simulink model "dtmf"  (R2018b)
settings: Solver=VariableStepAuto  StartTime=0.0  StopTime=105  RelTol=1e-3
libraries: dspsrcs4 x35, simulink x24, dspbuff3 x14, dspsigops x3, dspswit3 x1
settings Model: Creator=sajan.gict16  LastModifiedBy=srg
settings DebuggingCC: LibraryContextMissingDiagnostic=none
settings SFSimCC: SimUseLocalCustomCode=off
settings RTWCC: RTWUseLocalCustomCode=off

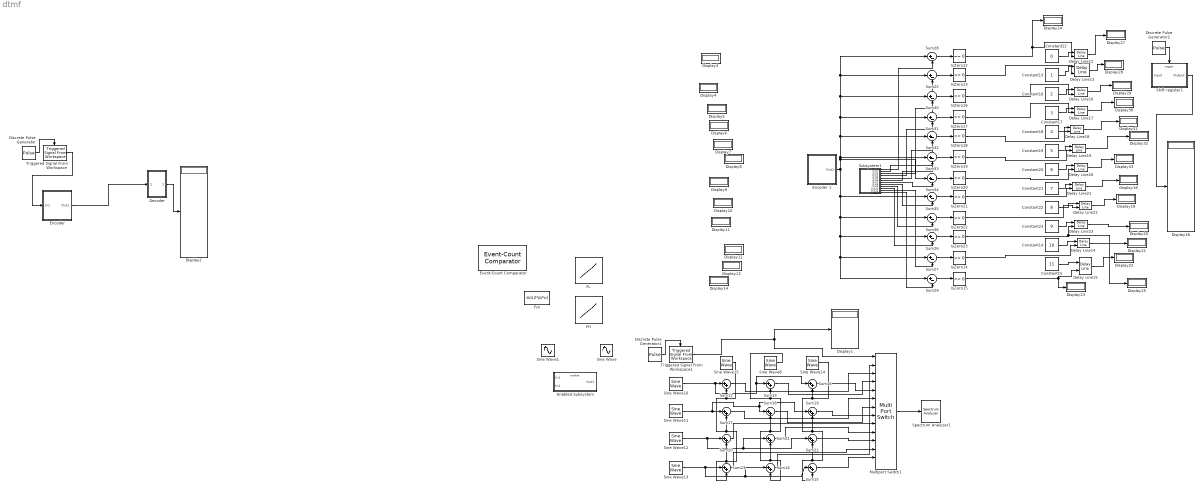
== system dtmf ==
  Constant12 : Constant  Value=0  SampleTime=1/12000
  Constant13 : Constant  SampleTime=1/12000
  Constant14 : Constant  Value=10  SampleTime=1/12000
  Constant15 : Constant  Value=11  SampleTime=1/12000
  Constant16 : Constant  Value=2  SampleTime=1/12000
  Constant17 : Constant  Value=3  SampleTime=1/12000
  Constant18 : Constant  Value=4  SampleTime=1/12000
  Constant19 : Constant  Value=5  SampleTime=1/12000
  Constant20 : Constant  Value=6  SampleTime=1/12000
  Constant21 : Constant  Value=7  SampleTime=1/12000
  Constant22 : Constant  Value=8  SampleTime=1/12000
  Constant23 : Constant  Value=9  SampleTime=1/12000
  "Decoder " : Subsystem
  Delay Line12 : dspbuff3/Delay Line  siz=3  ic=0  directfeed=off  enable_output=on  hold_output=on  OutputFrames=off
      settings: SourceProductName=DSP System Toolbox  SourceProductBaseCode=DS
  Delay Line13 : dspbuff3/Delay Line  siz=2  ic=0  directfeed=off  enable_output=on  hold_output=on  OutputFrames=off
      settings: SourceProductName=DSP System Toolbox  SourceProductBaseCode=DS
  Delay Line14 : dspbuff3/Delay Line  siz=2  ic=0  directfeed=on  enable_output=on  hold_output=on  OutputFrames=off
      settings: SourceProductName=DSP System Toolbox  SourceProductBaseCode=DS
  Delay Line15 : dspbuff3/Delay Line  siz=2  ic=0  directfeed=on  enable_output=on  hold_output=on  OutputFrames=off
      settings: SourceProductName=DSP System Toolbox  SourceProductBaseCode=DS
  Delay Line16 : dspbuff3/Delay Line  siz=3  ic=0  directfeed=off  enable_output=on  hold_output=on  OutputFrames=off
      settings: SourceProductName=DSP System Toolbox  SourceProductBaseCode=DS
  Delay Line17 : dspbuff3/Delay Line  siz=3  ic=0  directfeed=off  enable_output=on  hold_output=off  OutputFrames=off
      settings: SourceProductName=DSP System Toolbox  SourceProductBaseCode=DS
  Delay Line{18..22} (5 alike) : dspbuff3/Delay Line  siz=2  ic=0  directfeed=on  enable_output=on  hold_output=off  OutputFrames=off
      settings: SourceProductName=DSP System Toolbox  SourceProductBaseCode=DS
  Delay Line23 : dspbuff3/Delay Line  siz=2  ic=0  directfeed=off  enable_output=on  hold_output=off  OutputFrames=off
      settings: SourceProductName=DSP System Toolbox  SourceProductBaseCode=DS
  Discrete Pulse Generator : DiscretePulseGenerator  SampleTime=5
  Discrete Pulse Generator1 : DiscretePulseGenerator  SampleTime=5
  Discrete Pulse Generator2 : DiscretePulseGenerator  SampleTime=5
  Display{1..14,18..33} (30 alike) : Display
  Enabled Subsystem : Subsystem  TreatAsAtomicUnit=on
  "Encoder " : Subsystem
  Encoder 1 : Subsystem
  Event-Count Comparator : dspswit3/Event-Count Comparator  Threshold=10
      settings: SourceProductName=DSP System Toolbox  SourceProductBaseCode=DS
  FH : Lookup_n-D  NumberOfTableDimensions=1  BreakpointsForDimension1=[0,1,2,3,4,5,6,7,8,9,10,11]  Table=[1336,1209,1336,1477,1209,1336,1477,1209,1336,1477,1209,1477]  InternalRulePriority=Speed  RndMeth=Simplest  InputSameDT=on
  "FL " : Lookup_n-D  NumberOfTableDimensions=1  BreakpointsForDimension1=[0,1,2,3,4,5,6,7,8,9,10,11]  Table=[941,697,697,697,770,770,770,852,852,852,941,941]  InternalRulePriority=Speed  RndMeth=Simplest  InputSameDT=on
  Fcn : Fcn  Expr=sin(2*pi*u)
  IsZero{12..23} (12 alike) : simulink/Logic and Bit Operations/Compare To Zero  relop===  OutDataTypeStr=boolean
  Multiport Switch1 : MultiPortSwitch  DataPortOrder=Zero-based contiguous  Inputs=12  DataPortIndices={1,2,3,4,5,6,7,8,9,10,0,11}  DataPortForDefault=Additional data port  DiagnosticForDefault=Warning  zeroidx=on
  Shift register1 : Subsystem  TreatAsAtomicUnit=on
  Sine Wave : Sin  SampleTime=0
  Sine Wave1 : Sin  SampleTime=0
  Sine Wave10 : dspsrcs4/Sine Wave  Amplitude=1  Frequency=697  Phase=0  SampleMode=Discrete  OutComplex=Real  CompMethod=Trigonometric fcn  TableSize=Speed  SampleTime=1/12000  SamplesPerFrame=1  ResetState=Restart at time zero  OutputFrames=off  dataType=double  wordLen=16  udDataType=sfix(16)  fracBitsMode=Best precision  numFracBits=15  OutDataTypeStr=double  LastOutDataTypeStr=double
  Sine Wave11 : dspsrcs4/Sine Wave  Amplitude=1  Frequency=770  Phase=0  SampleMode=Discrete  OutComplex=Real  CompMethod=Trigonometric fcn  TableSize=Speed  SampleTime=1/12000  SamplesPerFrame=1  ResetState=Restart at time zero  OutputFrames=off  dataType=double  wordLen=16  udDataType=sfix(16)  fracBitsMode=Best precision  numFracBits=15  OutDataTypeStr=double  LastOutDataTypeStr=double
  Sine Wave12 : dspsrcs4/Sine Wave  Amplitude=1  Frequency=852  Phase=0  SampleMode=Discrete  OutComplex=Real  CompMethod=Trigonometric fcn  TableSize=Speed  SampleTime=1/12000  SamplesPerFrame=1  ResetState=Restart at time zero  OutputFrames=off  dataType=double  wordLen=16  udDataType=sfix(16)  fracBitsMode=Best precision  numFracBits=15  OutDataTypeStr=double  LastOutDataTypeStr=double
  Sine Wave13 : dspsrcs4/Sine Wave  Amplitude=1  Frequency=941  Phase=0  SampleMode=Discrete  OutComplex=Real  CompMethod=Trigonometric fcn  TableSize=Speed  SampleTime=1/12000  SamplesPerFrame=1  ResetState=Restart at time zero  OutputFrames=off  dataType=double  wordLen=16  udDataType=sfix(16)  fracBitsMode=Best precision  numFracBits=15  OutDataTypeStr=double  LastOutDataTypeStr=double
  Sine Wave14 : dspsrcs4/Sine Wave  Amplitude=1  Frequency=1477  Phase=0  SampleMode=Discrete  OutComplex=Real  CompMethod=Trigonometric fcn  TableSize=Speed  SampleTime=1/12000  SamplesPerFrame=1  ResetState=Restart at time zero  OutputFrames=off  dataType=double  wordLen=16  udDataType=sfix(16)  fracBitsMode=Best precision  numFracBits=15  OutDataTypeStr=double  LastOutDataTypeStr=double
  Sine Wave15 : dspsrcs4/Sine Wave  Amplitude=1  Frequency=1209  Phase=0  SampleMode=Discrete  OutComplex=Real  CompMethod=Trigonometric fcn  TableSize=Speed  SampleTime=1/12000  SamplesPerFrame=1  ResetState=Restart at time zero  OutputFrames=off  dataType=double  wordLen=16  udDataType=sfix(16)  fracBitsMode=Best precision  numFracBits=15  OutDataTypeStr=double  LastOutDataTypeStr=double
  Sine Wave8 : dspsrcs4/Sine Wave  Amplitude=1  Frequency=1336  Phase=0  SampleMode=Discrete  OutComplex=Real  CompMethod=Trigonometric fcn  TableSize=Speed  SampleTime=1/12000  SamplesPerFrame=1  ResetState=Restart at time zero  OutputFrames=off  dataType=double  wordLen=16  udDataType=sfix(16)  fracBitsMode=Best precision  numFracBits=15  OutDataTypeStr=double  LastOutDataTypeStr=double
  Spectrum Analyzer1 : SpectrumAnalyzer
  Subsystem1 : Subsystem
  Sum{12..23} (12 alike) : Sum  Inputs=|++
  Sum{25..36} (12 alike) : Sum  Inputs=|+-
  Triggered Signal From Workspace : dspsigops/Triggered Signal From Workspace  Signal=[0 2 0 8 7 6 5 4 9 10]  TriggerType=Rising edge  ic=0  SamplesPerFrame=1  OutputAfterFinalValue=Setting to zero  OutputFrames=off
      settings: SourceProductName=DSP System Toolbox  SourceProductBaseCode=DS
  Triggered Signal From Workspace1 : dspsigops/Triggered Signal From Workspace  Signal=[1 2 3 8 7 6 5 4 9 10]  TriggerType=Rising edge  ic=0  SamplesPerFrame=1  OutputAfterFinalValue=Setting to zero  OutputFrames=off
      settings: SourceProductName=DSP System Toolbox  SourceProductBaseCode=DS
  wires:
  Sum16/1 -> Multiport Switch1/5
  Sum19/1 -> Multiport Switch1/8
  Sum18/1 -> Multiport Switch1/7
  Sum23/1 -> Multiport Switch1/12
  Sine Wave14/1 -> Sum15/2, Sum22/2, Sum19/2, Sum16/2
  Sum15/1 -> Multiport Switch1/13
  Sum21/1 -> Multiport Switch1/10
  Sum12/1 -> Multiport Switch1/3
  Sum17/1 -> Multiport Switch1/6
  Triggered Signal From Workspace1/1 -> Multiport Switch1/1, Display1/1
  Multiport Switch1/1 -> Spectrum Analyzer1/1
  Sum13/1 -> Multiport Switch1/4
  Sine Wave15/1 -> Sum23/2, Sum20/2, Sum17/2, Sum12/2
  Sum20/1 -> Multiport Switch1/9
  Sum14/1 -> Multiport Switch1/2
  Sine Wave8/1 -> Sum14/2, Sum21/2, Sum18/2, Sum13/2
  Sine Wave13/1 -> Sum14/1, Sum15/1, Sum23/1
  Sine Wave11/1 -> Sum18/1, Sum19/1, Sum17/1
  Sine Wave12/1 -> Sum22/1, Sum21/1, Sum20/1
  Sine Wave10/1 -> Sum16/1, Sum13/1, Sum12/1
  Discrete Pulse Generator1/1 -> Triggered Signal From Workspace1/Trigger
  Sum22/1 -> Multiport Switch1/11
  Subsystem1/12(Out12) -> Sum29/2
  Subsystem1/10(Out10) -> Sum26/2
  Subsystem1/9(Out9) -> Sum36/2
  Subsystem1/8(Out8) -> Sum35/2
  Sum28/1 -> IsZero12/1
  IsZero19/1 -> Delay Line19/2
  Constant14/1 -> Delay Line14/1
  IsZero21/1 -> Delay Line21/2
  Subsystem1/4(Out4) -> Sum31/2
  Subsystem1/3(Out3) -> Sum30/2
  Subsystem1/2(Out2) -> Sum25/2
  Subsystem1/7(Out7) -> Sum34/2
  Subsystem1/6(Out6) -> Sum33/2
  Subsystem1/5(Out5) -> Sum32/2
  Sum26/1 -> IsZero23/1
  Sum35/1 -> IsZero21/1
  Sum29/1 -> IsZero15/1
  Sum36/1 -> IsZero22/1
  Sum27/1 -> IsZero14/1
  Subsystem1/1(Out1) -> Sum28/2
  IsZero14/1 -> Delay Line14/2
  Delay Line15/1 -> Display22/1
  Delay Line20/1 -> Display33/1
  Sum31/1 -> IsZero17/1
  Constant18/1 -> Delay Line18/1
  Discrete Pulse Generator2/1 -> Shift register1/Trigger
  IsZero16/1 -> Delay Line16/2
  Encoder 1/1(Out1) -> Sum29/1, Sum27/1, Sum26/1, Sum36/1, Sum35/1, Sum34/1, Sum32/1, Sum28/1, Sum25/1, Sum30/1, Sum31/1, Sum33/1
  IsZero18/1 -> Delay Line18/2
  Sum34/1 -> IsZero20/1
  Delay Line18/1 -> Display31/1
  IsZero20/1 -> Delay Line20/2
  Constant23/1 -> Delay Line23/1
  Constant21/1 -> Delay Line21/1
  IsZero12/1 -> Display24/1, Delay Line12/2
  Delay Line13/1 -> Display28/1
  Constant19/1 -> Delay Line19/1
  IsZero23/1 -> Display25/1, Delay Line23/2
  IsZero13/1 -> Delay Line13/2
  Delay Line14/1 -> Display21/1
  IsZero22/1 -> Delay Line22/2
  IsZero17/1 -> Delay Line17/2
  IsZero15/1 -> Delay Line15/2, Display23/1
  Delay Line21/1 -> Display18/1
  Delay Line22/1 -> Display19/1
  Constant22/1 -> Delay Line22/1
  Delay Line16/1 -> Display29/1
  Constant20/1 -> Delay Line20/1
  Constant17/1 -> Delay Line17/1
  Constant15/1 -> Delay Line15/1
  Constant12/1 -> Delay Line12/1
  Constant16/1 -> Delay Line16/1
  Delay Line17/1 -> Display30/1
  Subsystem1/11(Out11) -> Sum27/2
  Sum32/1 -> IsZero18/1
  Delay Line19/1 -> Display32/1
  Sum30/1 -> IsZero16/1
  Sum25/1 -> IsZero13/1
  Delay Line23/1 -> Display20/1
  Constant13/1 -> Delay Line13/1
  Shift register1/1(Output) -> Display26/1
  Sum33/1 -> IsZero19/1
  Delay Line12/1 -> Display27/1
  ? -> Display6/1
  ? -> Display9/1
  ? -> Display8/1
  ? -> Display10/1
  ? -> Display11/1
  ? -> Display5/1
  ? -> Display12/1
  ? -> Display7/1
  ? -> Display3/1
  ? -> Display14/1
  ? -> Display13/1
  "Encoder "/1(Out1) -> "Decoder "/1(In1)
  "Decoder "/1(Out1) -> Display2/1
  Discrete Pulse Generator/1 -> Triggered Signal From Workspace/Trigger
  Triggered Signal From Workspace/1 -> "Encoder "/1(In1)

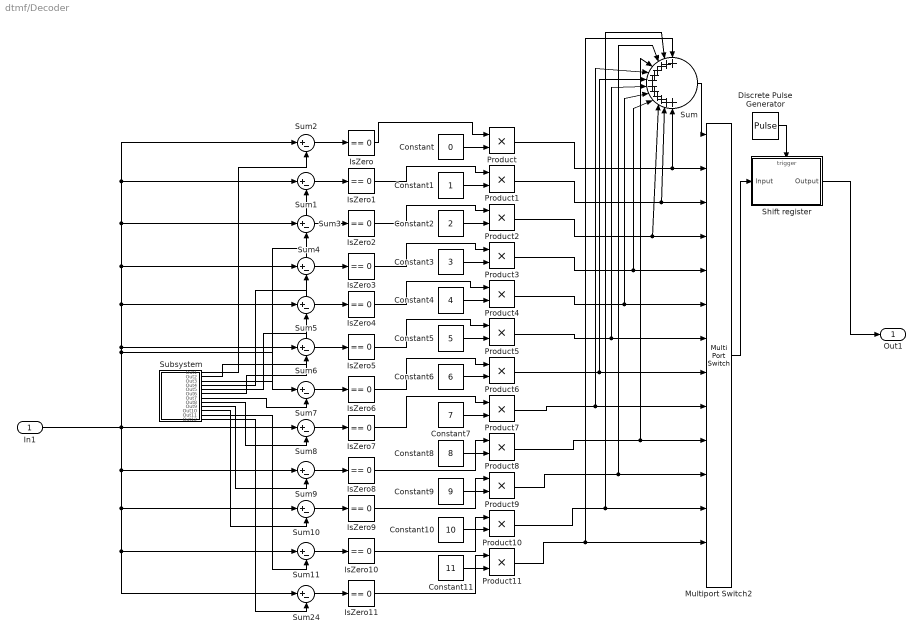
== system dtmf/Decoder  ==
  In1 : Inport
  Constant : Constant  Value=0  SampleTime=1/12000
  Constant1 : Constant  SampleTime=1/12000
  Constant10 : Constant  Value=10  SampleTime=1/12000
  Constant11 : Constant  Value=11  SampleTime=1/12000
  Constant2 : Constant  Value=2  SampleTime=1/12000
  Constant3 : Constant  Value=3  SampleTime=1/12000
  Constant4 : Constant  Value=4  SampleTime=1/12000
  Constant5 : Constant  Value=5  SampleTime=1/12000
  Constant6 : Constant  Value=6  SampleTime=1/12000
  Constant7 : Constant  Value=7  SampleTime=1/12000
  Constant8 : Constant  Value=8  SampleTime=1/12000
  Constant9 : Constant  Value=9  SampleTime=1/12000
  Discrete Pulse Generator : DiscretePulseGenerator  SampleTime=5
  IsZero{,1..11} (12 alike) : simulink/Logic and Bit Operations/Compare To Zero  relop===  OutDataTypeStr=boolean
  Multiport Switch2 : MultiPortSwitch  DataPortOrder=Zero-based contiguous  Inputs=12  DataPortIndices={1,2,3,4,5,6,7,8,9,10,0,11}  DataPortForDefault=Additional data port  DiagnosticForDefault=Warning  zeroidx=on
  Product{,1..11} (12 alike) : Product
  Shift register : Subsystem  TreatAsAtomicUnit=on
  Subsystem : Subsystem
  Sum : Sum  Inputs=12
  Sum{1..11,24} (12 alike) : Sum  Inputs=|+-
  Out1 : Outport
  wires:
  IsZero7/1 -> Product7/1
  Subsystem/6(Out6) -> Sum6/2
  Product7/1 -> Sum/5, Multiport Switch2/9
  Constant1/1 -> Product1/2
  Sum6/1 -> IsZero5/1
  Sum7/1 -> IsZero6/1
  Discrete Pulse Generator/1 -> Shift register/Trigger
  Product3/1 -> Sum/9, Multiport Switch2/5
  Sum3/1 -> IsZero2/1
  Product8/1 -> Sum/4, Multiport Switch2/10
  In1/1 -> Sum7/1, Sum5/1, Sum2/1, Sum1/1, Sum3/1, Sum4/1, Sum6/1, Sum24/1, Sum11/1, Sum10/1, Sum9/1, Sum8/1
  Sum1/1 -> IsZero1/1
  Multiport Switch2/1 -> Shift register/1(Input)
  Constant11/1 -> Product11/2
  Product5/1 -> Sum/7, Multiport Switch2/7
  Sum4/1 -> IsZero3/1
  Subsystem/9(Out9) -> Sum9/2
  Subsystem/4(Out4) -> Sum4/2
  Constant3/1 -> Product3/2
  Sum24/1 -> IsZero11/1
  Sum5/1 -> IsZero4/1
  Product2/1 -> Sum/10, Multiport Switch2/4
  IsZero9/1 -> Product9/1
  Product10/1 -> Multiport Switch2/12, Sum/2
  Constant10/1 -> Product10/2
  Constant5/1 -> Product5/2
  Constant7/1 -> Product7/2
  Sum2/1 -> IsZero/1
  IsZero4/1 -> Product4/1
  IsZero10/1 -> Product10/1
  Constant8/1 -> Product8/2
  Product4/1 -> Sum/8, Multiport Switch2/6
  Product1/1 -> Sum/11, Multiport Switch2/3
  Product11/1 -> Multiport Switch2/13, Sum/1
  Sum/1 -> Multiport Switch2/1
  Product/1 -> Sum/12, Multiport Switch2/2
  IsZero11/1 -> Product11/1
  IsZero/1 -> Product/1
  Subsystem/5(Out5) -> Sum5/2
  IsZero6/1 -> Product6/1
  Subsystem/1(Out1) -> Sum2/2
  Constant/1 -> Product/2
  IsZero1/1 -> Product1/1
  Constant9/1 -> Product9/2
  Product9/1 -> Multiport Switch2/11, Sum/3
  IsZero3/1 -> Product3/1
  Subsystem/12(Out12) -> Sum24/2
  Constant2/1 -> Product2/2
  Constant6/1 -> Product6/2
  Product6/1 -> Sum/6, Multiport Switch2/8
  Subsystem/10(Out10) -> Sum10/2
  Constant4/1 -> Product4/2
  IsZero5/1 -> Product5/1
  IsZero8/1 -> Product8/1
  Sum11/1 -> IsZero10/1
  Sum9/1 -> IsZero8/1
  Sum8/1 -> IsZero7/1
  Sum10/1 -> IsZero9/1
  Subsystem/8(Out8) -> Sum8/2
  Subsystem/7(Out7) -> Sum7/2
  Subsystem/2(Out2) -> Sum1/2
  Subsystem/3(Out3) -> Sum3/2
  Subsystem/11(Out11) -> Sum11/2
  IsZero2/1 -> Product2/1
  Shift register/1(Output) -> Out1/1

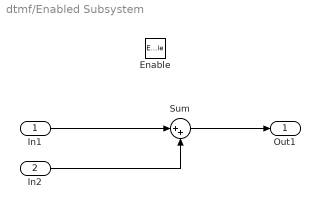
== system dtmf/Enabled Subsystem ==
  In1 : Inport
  In2 : Inport  Port=2
  Enable : EnablePort
  Sum : Sum  Inputs=|++
  Out1 : Outport
  wires:
  In1/1 -> Sum/1
  In2/1 -> Sum/2
  Sum/1 -> Out1/1

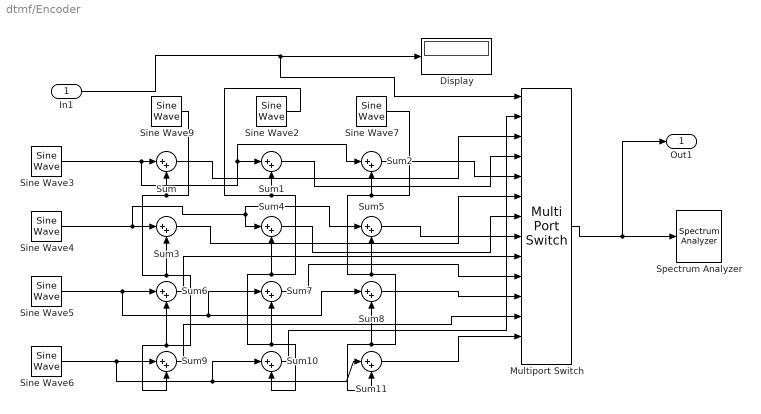
== system dtmf/Encoder  ==
  In1 : Inport
  Display : Display
  Multiport Switch : MultiPortSwitch  DataPortOrder=Zero-based contiguous  Inputs=12  DataPortIndices={1,2,3,4,5,6,7,8,9,10,0,11}  DataPortForDefault=Additional data port  DiagnosticForDefault=Warning  zeroidx=on
  Sine Wave2 : dspsrcs4/Sine Wave  Amplitude=1  Frequency=1336  Phase=0  SampleMode=Discrete  OutComplex=Real  CompMethod=Trigonometric fcn  TableSize=Speed  SampleTime=1/12000  SamplesPerFrame=1  ResetState=Restart at time zero  OutputFrames=off  dataType=double  wordLen=16  udDataType=sfix(16)  fracBitsMode=Best precision  numFracBits=15  OutDataTypeStr=double  LastOutDataTypeStr=double
  Sine Wave3 : dspsrcs4/Sine Wave  Amplitude=1  Frequency=697  Phase=0  SampleMode=Discrete  OutComplex=Real  CompMethod=Trigonometric fcn  TableSize=Speed  SampleTime=1/12000  SamplesPerFrame=1  ResetState=Restart at time zero  OutputFrames=off  dataType=double  wordLen=16  udDataType=sfix(16)  fracBitsMode=Best precision  numFracBits=15  OutDataTypeStr=double  LastOutDataTypeStr=double
  Sine Wave4 : dspsrcs4/Sine Wave  Amplitude=1  Frequency=770  Phase=0  SampleMode=Discrete  OutComplex=Real  CompMethod=Trigonometric fcn  TableSize=Speed  SampleTime=1/12000  SamplesPerFrame=1  ResetState=Restart at time zero  OutputFrames=off  dataType=double  wordLen=16  udDataType=sfix(16)  fracBitsMode=Best precision  numFracBits=15  OutDataTypeStr=double  LastOutDataTypeStr=double
  Sine Wave5 : dspsrcs4/Sine Wave  Amplitude=1  Frequency=852  Phase=0  SampleMode=Discrete  OutComplex=Real  CompMethod=Trigonometric fcn  TableSize=Speed  SampleTime=1/12000  SamplesPerFrame=1  ResetState=Restart at time zero  OutputFrames=off  dataType=double  wordLen=16  udDataType=sfix(16)  fracBitsMode=Best precision  numFracBits=15  OutDataTypeStr=double  LastOutDataTypeStr=double
  Sine Wave6 : dspsrcs4/Sine Wave  Amplitude=1  Frequency=941  Phase=0  SampleMode=Discrete  OutComplex=Real  CompMethod=Trigonometric fcn  TableSize=Speed  SampleTime=1/12000  SamplesPerFrame=1  ResetState=Restart at time zero  OutputFrames=off  dataType=double  wordLen=16  udDataType=sfix(16)  fracBitsMode=Best precision  numFracBits=15  OutDataTypeStr=double  LastOutDataTypeStr=double
  Sine Wave7 : dspsrcs4/Sine Wave  Amplitude=1  Frequency=1477  Phase=0  SampleMode=Discrete  OutComplex=Real  CompMethod=Trigonometric fcn  TableSize=Speed  SampleTime=1/12000  SamplesPerFrame=1  ResetState=Restart at time zero  OutputFrames=off  dataType=double  wordLen=16  udDataType=sfix(16)  fracBitsMode=Best precision  numFracBits=15  OutDataTypeStr=double  LastOutDataTypeStr=double
  Sine Wave9 : dspsrcs4/Sine Wave  Amplitude=1  Frequency=1209  Phase=0  SampleMode=Discrete  OutComplex=Real  CompMethod=Trigonometric fcn  TableSize=Speed  SampleTime=1/12000  SamplesPerFrame=1  ResetState=Restart at time zero  OutputFrames=off  dataType=double  wordLen=16  udDataType=sfix(16)  fracBitsMode=Best precision  numFracBits=15  OutDataTypeStr=double  LastOutDataTypeStr=double
  Spectrum Analyzer : SpectrumAnalyzer
  Sum{,1..11} (12 alike) : Sum  Inputs=|++
  Out1 : Outport
  wires:
  Sine Wave2/1 -> Sum10/2, Sum7/2, Sum4/2, Sum1/2
  Sine Wave6/1 -> Sum10/1, Sum11/1, Sum9/1
  Sine Wave7/1 -> Sum11/2, Sum8/2, Sum5/2, Sum2/2
  Sum8/1 -> Multiport Switch/11
  Sum10/1 -> Multiport Switch/2
  Sine Wave3/1 -> Sum2/1, Sum1/1, Sum/1
  Sum9/1 -> Multiport Switch/12
  Sine Wave4/1 -> Sum4/1, Sum5/1, Sum3/1
  Sine Wave5/1 -> Sum8/1, Sum7/1, Sum6/1
  Sum6/1 -> Multiport Switch/9
  Sum3/1 -> Multiport Switch/6
  Sine Wave9/1 -> Sum9/2, Sum6/2, Sum3/2, Sum/2
  Sum1/1 -> Multiport Switch/4
  Multiport Switch/1 -> Out1/1, Spectrum Analyzer/1
  In1/1 -> Multiport Switch/1, Display/1
  Sum/1 -> Multiport Switch/3
  Sum7/1 -> Multiport Switch/10
  Sum11/1 -> Multiport Switch/13
  Sum4/1 -> Multiport Switch/7
  Sum5/1 -> Multiport Switch/8
  Sum2/1 -> Multiport Switch/5

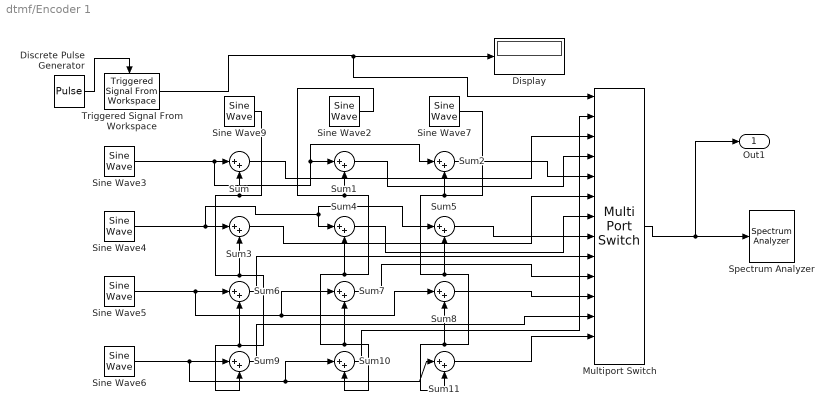
== system dtmf/Encoder 1 ==
  Discrete Pulse Generator : DiscretePulseGenerator  SampleTime=5
  Display : Display
  Multiport Switch : MultiPortSwitch  DataPortOrder=Zero-based contiguous  Inputs=12  DataPortIndices={1,2,3,4,5,6,7,8,9,10,0,11}  DataPortForDefault=Additional data port  DiagnosticForDefault=Warning  zeroidx=on
  Sine Wave2 : dspsrcs4/Sine Wave  Amplitude=1  Frequency=1336  Phase=0  SampleMode=Discrete  OutComplex=Real  CompMethod=Trigonometric fcn  TableSize=Speed  SampleTime=1/12000  SamplesPerFrame=1  ResetState=Restart at time zero  OutputFrames=off  dataType=double  wordLen=16  udDataType=sfix(16)  fracBitsMode=Best precision  numFracBits=15  OutDataTypeStr=double  LastOutDataTypeStr=double
  Sine Wave3 : dspsrcs4/Sine Wave  Amplitude=1  Frequency=697  Phase=0  SampleMode=Discrete  OutComplex=Real  CompMethod=Trigonometric fcn  TableSize=Speed  SampleTime=1/12000  SamplesPerFrame=1  ResetState=Restart at time zero  OutputFrames=off  dataType=double  wordLen=16  udDataType=sfix(16)  fracBitsMode=Best precision  numFracBits=15  OutDataTypeStr=double  LastOutDataTypeStr=double
  Sine Wave4 : dspsrcs4/Sine Wave  Amplitude=1  Frequency=770  Phase=0  SampleMode=Discrete  OutComplex=Real  CompMethod=Trigonometric fcn  TableSize=Speed  SampleTime=1/12000  SamplesPerFrame=1  ResetState=Restart at time zero  OutputFrames=off  dataType=double  wordLen=16  udDataType=sfix(16)  fracBitsMode=Best precision  numFracBits=15  OutDataTypeStr=double  LastOutDataTypeStr=double
  Sine Wave5 : dspsrcs4/Sine Wave  Amplitude=1  Frequency=852  Phase=0  SampleMode=Discrete  OutComplex=Real  CompMethod=Trigonometric fcn  TableSize=Speed  SampleTime=1/12000  SamplesPerFrame=1  ResetState=Restart at time zero  OutputFrames=off  dataType=double  wordLen=16  udDataType=sfix(16)  fracBitsMode=Best precision  numFracBits=15  OutDataTypeStr=double  LastOutDataTypeStr=double
  Sine Wave6 : dspsrcs4/Sine Wave  Amplitude=1  Frequency=941  Phase=0  SampleMode=Discrete  OutComplex=Real  CompMethod=Trigonometric fcn  TableSize=Speed  SampleTime=1/12000  SamplesPerFrame=1  ResetState=Restart at time zero  OutputFrames=off  dataType=double  wordLen=16  udDataType=sfix(16)  fracBitsMode=Best precision  numFracBits=15  OutDataTypeStr=double  LastOutDataTypeStr=double
  Sine Wave7 : dspsrcs4/Sine Wave  Amplitude=1  Frequency=1477  Phase=0  SampleMode=Discrete  OutComplex=Real  CompMethod=Trigonometric fcn  TableSize=Speed  SampleTime=1/12000  SamplesPerFrame=1  ResetState=Restart at time zero  OutputFrames=off  dataType=double  wordLen=16  udDataType=sfix(16)  fracBitsMode=Best precision  numFracBits=15  OutDataTypeStr=double  LastOutDataTypeStr=double
  Sine Wave9 : dspsrcs4/Sine Wave  Amplitude=1  Frequency=1209  Phase=0  SampleMode=Discrete  OutComplex=Real  CompMethod=Trigonometric fcn  TableSize=Speed  SampleTime=1/12000  SamplesPerFrame=1  ResetState=Restart at time zero  OutputFrames=off  dataType=double  wordLen=16  udDataType=sfix(16)  fracBitsMode=Best precision  numFracBits=15  OutDataTypeStr=double  LastOutDataTypeStr=double
  Spectrum Analyzer : SpectrumAnalyzer
  Sum{,1..11} (12 alike) : Sum  Inputs=|++
  Triggered Signal From Workspace : dspsigops/Triggered Signal From Workspace  Signal=[1 2 3 8 7 6 5 4 9 10]  TriggerType=Rising edge  ic=0  SamplesPerFrame=1  OutputAfterFinalValue=Setting to zero  OutputFrames=off
      settings: SourceProductName=DSP System Toolbox  SourceProductBaseCode=DS
  Out1 : Outport
  wires:
  Sine Wave2/1 -> Sum10/2, Sum7/2, Sum4/2, Sum1/2
  Sine Wave6/1 -> Sum10/1, Sum11/1, Sum9/1
  Sine Wave7/1 -> Sum11/2, Sum8/2, Sum5/2, Sum2/2
  Sum8/1 -> Multiport Switch/11
  Sum10/1 -> Multiport Switch/2
  Sine Wave3/1 -> Sum2/1, Sum1/1, Sum/1
  Sum9/1 -> Multiport Switch/12
  Discrete Pulse Generator/1 -> Triggered Signal From Workspace/Trigger
  Sine Wave4/1 -> Sum4/1, Sum5/1, Sum3/1
  Sine Wave5/1 -> Sum8/1, Sum7/1, Sum6/1
  Sum6/1 -> Multiport Switch/9
  Sum3/1 -> Multiport Switch/6
  Sine Wave9/1 -> Sum9/2, Sum6/2, Sum3/2, Sum/2
  Sum1/1 -> Multiport Switch/4
  Multiport Switch/1 -> Out1/1, Spectrum Analyzer/1
  Triggered Signal From Workspace/1 -> Multiport Switch/1, Display/1
  Sum/1 -> Multiport Switch/3
  Sum7/1 -> Multiport Switch/10
  Sum11/1 -> Multiport Switch/13
  Sum4/1 -> Multiport Switch/7
  Sum5/1 -> Multiport Switch/8
  Sum2/1 -> Multiport Switch/5

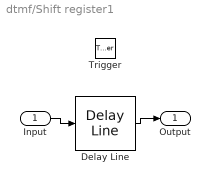
== system dtmf/Shift register1 ==
  Input : Inport
  Trigger : TriggerPort  VariantControl=Variant  ZeroCross=off
  Delay Line : dspbuff3/Delay Line  siz=11  ic=0  directfeed=on  enable_output=off  hold_output=off  OutputFrames=off
      settings: SourceProductName=DSP System Toolbox  SourceProductBaseCode=DS
  Output : Outport
  wires:
  Input/1 -> Delay Line/1
  Delay Line/1 -> Output/1

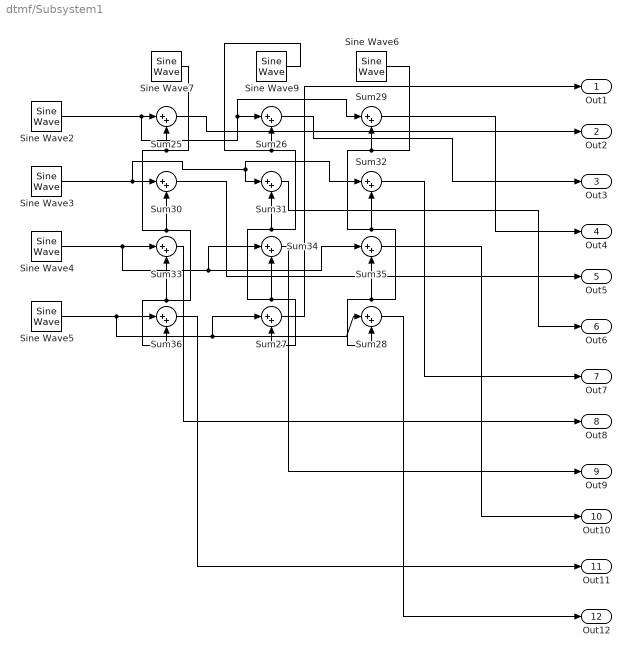
== system dtmf/Subsystem1 ==
  Sine Wave2 : dspsrcs4/Sine Wave  Amplitude=1  Frequency=697  Phase=0  SampleMode=Discrete  OutComplex=Real  CompMethod=Trigonometric fcn  TableSize=Speed  SampleTime=1/12000  SamplesPerFrame=1  ResetState=Restart at time zero  OutputFrames=off  dataType=double  wordLen=16  udDataType=sfix(16)  fracBitsMode=Best precision  numFracBits=15  OutDataTypeStr=double  LastOutDataTypeStr=double
  Sine Wave3 : dspsrcs4/Sine Wave  Amplitude=1  Frequency=770  Phase=0  SampleMode=Discrete  OutComplex=Real  CompMethod=Trigonometric fcn  TableSize=Speed  SampleTime=1/12000  SamplesPerFrame=1  ResetState=Restart at time zero  OutputFrames=off  dataType=double  wordLen=16  udDataType=sfix(16)  fracBitsMode=Best precision  numFracBits=15  OutDataTypeStr=double  LastOutDataTypeStr=double
  Sine Wave4 : dspsrcs4/Sine Wave  Amplitude=1  Frequency=852  Phase=0  SampleMode=Discrete  OutComplex=Real  CompMethod=Trigonometric fcn  TableSize=Speed  SampleTime=1/12000  SamplesPerFrame=1  ResetState=Restart at time zero  OutputFrames=off  dataType=double  wordLen=16  udDataType=sfix(16)  fracBitsMode=Best precision  numFracBits=15  OutDataTypeStr=double  LastOutDataTypeStr=double
  Sine Wave5 : dspsrcs4/Sine Wave  Amplitude=1  Frequency=941  Phase=0  SampleMode=Discrete  OutComplex=Real  CompMethod=Trigonometric fcn  TableSize=Speed  SampleTime=1/12000  SamplesPerFrame=1  ResetState=Restart at time zero  OutputFrames=off  dataType=double  wordLen=16  udDataType=sfix(16)  fracBitsMode=Best precision  numFracBits=15  OutDataTypeStr=double  LastOutDataTypeStr=double
  Sine Wave6 : dspsrcs4/Sine Wave  Amplitude=1  Frequency=1477  Phase=0  SampleMode=Discrete  OutComplex=Real  CompMethod=Trigonometric fcn  TableSize=Speed  SampleTime=1/12000  SamplesPerFrame=1  ResetState=Restart at time zero  OutputFrames=off  dataType=double  wordLen=16  udDataType=sfix(16)  fracBitsMode=Best precision  numFracBits=15  OutDataTypeStr=double  LastOutDataTypeStr=double
  Sine Wave7 : dspsrcs4/Sine Wave  Amplitude=1  Frequency=1209  Phase=0  SampleMode=Discrete  OutComplex=Real  CompMethod=Trigonometric fcn  TableSize=Speed  SampleTime=1/12000  SamplesPerFrame=1  ResetState=Restart at time zero  OutputFrames=off  dataType=double  wordLen=16  udDataType=sfix(16)  fracBitsMode=Best precision  numFracBits=15  OutDataTypeStr=double  LastOutDataTypeStr=double
  Sine Wave9 : dspsrcs4/Sine Wave  Amplitude=1  Frequency=1336  Phase=0  SampleMode=Discrete  OutComplex=Real  CompMethod=Trigonometric fcn  TableSize=Speed  SampleTime=1/12000  SamplesPerFrame=1  ResetState=Restart at time zero  OutputFrames=off  dataType=double  wordLen=16  udDataType=sfix(16)  fracBitsMode=Best precision  numFracBits=15  OutDataTypeStr=double  LastOutDataTypeStr=double
  Sum{25..36} (12 alike) : Sum  Inputs=|++
  Out1 : Outport
  Out2 : Outport  Port=2
  Out3 : Outport  Port=3
  Out4 : Outport  Port=4
  Out5 : Outport  Port=5
  Out6 : Outport  Port=6
  Out7 : Outport  Port=7
  Out8 : Outport  Port=8
  Out9 : Outport  Port=9
  Out10 : Outport  Port=10
  Out11 : Outport  Port=11
  Out12 : Outport  Port=12
  wires:
  Sum32/1 -> Out7/1
  Sine Wave4/1 -> Sum35/1, Sum34/1, Sum33/1
  Sum31/1 -> Out6/1
  Sum29/1 -> Out4/1
  Sine Wave6/1 -> Sum28/2, Sum35/2, Sum32/2, Sum29/2
  Sum26/1 -> Out3/1
  Sum27/1 -> Out1/1
  Sine Wave7/1 -> Sum36/2, Sum33/2, Sum30/2, Sum25/2
  Sine Wave3/1 -> Sum31/1, Sum32/1, Sum30/1
  Sine Wave9/1 -> Sum27/2, Sum34/2, Sum31/2, Sum26/2
  Sine Wave2/1 -> Sum29/1, Sum26/1, Sum25/1
  Sine Wave5/1 -> Sum27/1, Sum28/1, Sum36/1
  Sum25/1 -> Out2/1
  Sum28/1 -> Out12/1
  Sum33/1 -> Out8/1
  Sum34/1 -> Out9/1
  Sum35/1 -> Out10/1
  Sum36/1 -> Out11/1
  Sum30/1 -> Out5/1

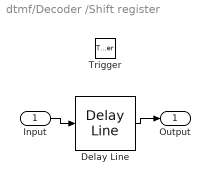
== system dtmf/Decoder /Shift register ==
  Input : Inport
  Trigger : TriggerPort  VariantControl=Variant  ZeroCross=off
  Delay Line : dspbuff3/Delay Line  siz=10  ic=0  directfeed=on  enable_output=off  hold_output=off  OutputFrames=off
      settings: SourceProductName=DSP System Toolbox  SourceProductBaseCode=DS
  Output : Outport
  wires:
  Input/1 -> Delay Line/1
  Delay Line/1 -> Output/1

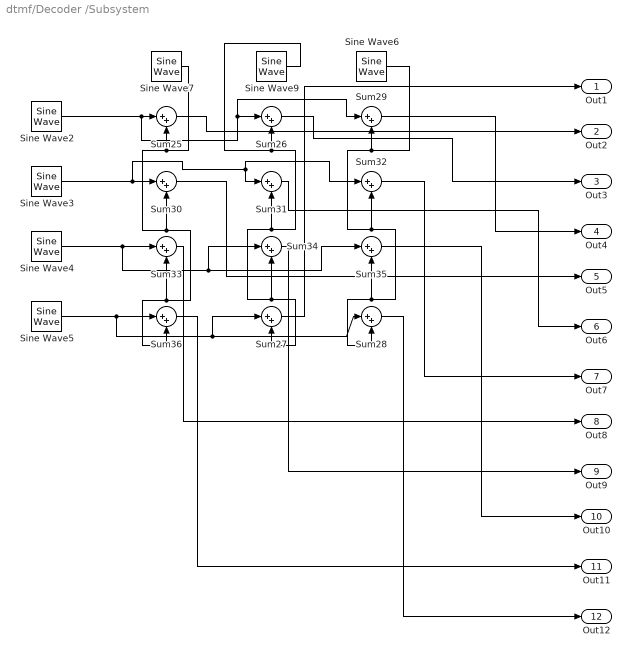
== system dtmf/Decoder /Subsystem ==
  Sine Wave2 : dspsrcs4/Sine Wave  Amplitude=1  Frequency=697  Phase=0  SampleMode=Discrete  OutComplex=Real  CompMethod=Trigonometric fcn  TableSize=Speed  SampleTime=1/12000  SamplesPerFrame=1  ResetState=Restart at time zero  OutputFrames=off  dataType=double  wordLen=16  udDataType=sfix(16)  fracBitsMode=Best precision  numFracBits=15  OutDataTypeStr=double  LastOutDataTypeStr=double
  Sine Wave3 : dspsrcs4/Sine Wave  Amplitude=1  Frequency=770  Phase=0  SampleMode=Discrete  OutComplex=Real  CompMethod=Trigonometric fcn  TableSize=Speed  SampleTime=1/12000  SamplesPerFrame=1  ResetState=Restart at time zero  OutputFrames=off  dataType=double  wordLen=16  udDataType=sfix(16)  fracBitsMode=Best precision  numFracBits=15  OutDataTypeStr=double  LastOutDataTypeStr=double
  Sine Wave4 : dspsrcs4/Sine Wave  Amplitude=1  Frequency=852  Phase=0  SampleMode=Discrete  OutComplex=Real  CompMethod=Trigonometric fcn  TableSize=Speed  SampleTime=1/12000  SamplesPerFrame=1  ResetState=Restart at time zero  OutputFrames=off  dataType=double  wordLen=16  udDataType=sfix(16)  fracBitsMode=Best precision  numFracBits=15  OutDataTypeStr=double  LastOutDataTypeStr=double
  Sine Wave5 : dspsrcs4/Sine Wave  Amplitude=1  Frequency=941  Phase=0  SampleMode=Discrete  OutComplex=Real  CompMethod=Trigonometric fcn  TableSize=Speed  SampleTime=1/12000  SamplesPerFrame=1  ResetState=Restart at time zero  OutputFrames=off  dataType=double  wordLen=16  udDataType=sfix(16)  fracBitsMode=Best precision  numFracBits=15  OutDataTypeStr=double  LastOutDataTypeStr=double
  Sine Wave6 : dspsrcs4/Sine Wave  Amplitude=1  Frequency=1477  Phase=0  SampleMode=Discrete  OutComplex=Real  CompMethod=Trigonometric fcn  TableSize=Speed  SampleTime=1/12000  SamplesPerFrame=1  ResetState=Restart at time zero  OutputFrames=off  dataType=double  wordLen=16  udDataType=sfix(16)  fracBitsMode=Best precision  numFracBits=15  OutDataTypeStr=double  LastOutDataTypeStr=double
  Sine Wave7 : dspsrcs4/Sine Wave  Amplitude=1  Frequency=1209  Phase=0  SampleMode=Discrete  OutComplex=Real  CompMethod=Trigonometric fcn  TableSize=Speed  SampleTime=1/12000  SamplesPerFrame=1  ResetState=Restart at time zero  OutputFrames=off  dataType=double  wordLen=16  udDataType=sfix(16)  fracBitsMode=Best precision  numFracBits=15  OutDataTypeStr=double  LastOutDataTypeStr=double
  Sine Wave9 : dspsrcs4/Sine Wave  Amplitude=1  Frequency=1336  Phase=0  SampleMode=Discrete  OutComplex=Real  CompMethod=Trigonometric fcn  TableSize=Speed  SampleTime=1/12000  SamplesPerFrame=1  ResetState=Restart at time zero  OutputFrames=off  dataType=double  wordLen=16  udDataType=sfix(16)  fracBitsMode=Best precision  numFracBits=15  OutDataTypeStr=double  LastOutDataTypeStr=double
  Sum{25..36} (12 alike) : Sum  Inputs=|++
  Out1 : Outport
  Out2 : Outport  Port=2
  Out3 : Outport  Port=3
  Out4 : Outport  Port=4
  Out5 : Outport  Port=5
  Out6 : Outport  Port=6
  Out7 : Outport  Port=7
  Out8 : Outport  Port=8
  Out9 : Outport  Port=9
  Out10 : Outport  Port=10
  Out11 : Outport  Port=11
  Out12 : Outport  Port=12
  wires:
  Sum32/1 -> Out7/1
  Sine Wave4/1 -> Sum35/1, Sum34/1, Sum33/1
  Sum31/1 -> Out6/1
  Sum29/1 -> Out4/1
  Sine Wave6/1 -> Sum28/2, Sum35/2, Sum32/2, Sum29/2
  Sum26/1 -> Out3/1
  Sum27/1 -> Out1/1
  Sine Wave7/1 -> Sum36/2, Sum33/2, Sum30/2, Sum25/2
  Sine Wave3/1 -> Sum31/1, Sum32/1, Sum30/1
  Sine Wave9/1 -> Sum27/2, Sum34/2, Sum31/2, Sum26/2
  Sine Wave2/1 -> Sum29/1, Sum26/1, Sum25/1
  Sine Wave5/1 -> Sum27/1, Sum28/1, Sum36/1
  Sum25/1 -> Out2/1
  Sum28/1 -> Out12/1
  Sum33/1 -> Out8/1
  Sum34/1 -> Out9/1
  Sum35/1 -> Out10/1
  Sum36/1 -> Out11/1
  Sum30/1 -> Out5/1
